simulink model "tempE"  (Simulink 6.1)
settings: Solver=ode3  StartTime=0.0  StopTime=5  FixedStep=0.1  RelTol=1e-3
libraries: simulink x5
settings Model: LastModifiedBy=okawa
settings DebuggingCC: SolverPrmCheckMsg=warning

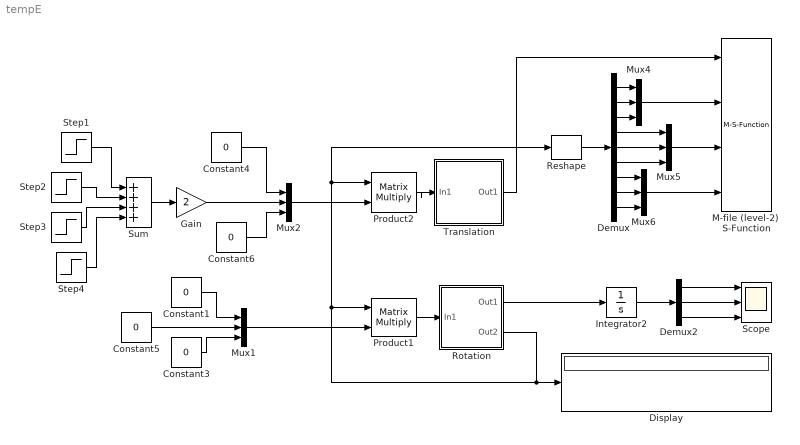
== system tempE ==
  Constant{1,3..6} (5 alike) : Constant  Value=0
  Demux : Demux  Outputs=9
  Demux2 : Demux  Outputs=3
  Display : Display
  Gain : Gain  Gain=2
  Integrator2 : Integrator
  M-file (level-2)  S-Function : M-S-Function  MFile=graphShip
  Mux{1..2,4..6} (5 alike) : Mux  Inputs=3
  Product1 : Product  Multiplication=Matrix(*)  RndMeth=Zero
  Product2 : Product  Multiplication=Matrix(*)  RndMeth=Zero
  Reshape : simulink/Math Operations/Reshape  OutputDimensionality=1-D array  OutputDimensions=[1,1]
  Rotation : Subsystem
  Scope : Scope  NumInputPorts=3
      settings: YMin=-5~-5~-5  YMax=5~5~5
  Step1 : Step  SampleTime=0
  Step2 : Step  Time=2  After=-2  SampleTime=0
  Step3 : Step  Time=4  After=2  SampleTime=0
  Step4 : Step  Time=5  After=-1  SampleTime=0
  Sum : Sum  Inputs=++++
  Translation : Subsystem
  wires:
  Demux/1 -> Mux4/1
  Demux/2 -> Mux4/2
  Demux/3 -> Mux4/3
  Demux/4 -> Mux5/1
  Demux/5 -> Mux5/2
  Demux/6 -> Mux5/3
  Demux/7 -> Mux6/1
  Demux/8 -> Mux6/2
  Demux/9 -> Mux6/3
  Rotation/1(Out1) -> Integrator2/1
  Rotation/2(Out2) -> Display/1, Product1/1, Reshape/1, Product2/1
  Product2/1 -> Translation/1(In1)
  Integrator2/1 -> Demux2/1
  Demux2/1 -> Scope/1
  Demux2/2 -> Scope/2
  Demux2/3 -> Scope/3
  Product1/1 -> Rotation/1(In1)
  Translation/1(Out1) -> M-file (level-2)  S-Function/1
  Reshape/1 -> Demux/1
  Mux2/1 -> Product2/2
  Step1/1 -> Sum/1
  Step2/1 -> Sum/2
  Step4/1 -> Sum/4
  Constant6/1 -> Mux2/3
  Step3/1 -> Sum/3
  Constant4/1 -> Mux2/1
  Sum/1 -> Gain/1
  Gain/1 -> Mux2/2
  Constant3/1 -> Mux1/3
  Constant5/1 -> Mux1/2
  Mux1/1 -> Product1/2
  Mux4/1 -> M-file (level-2)  S-Function/2
  Mux5/1 -> M-file (level-2)  S-Function/3
  Mux6/1 -> M-file (level-2)  S-Function/4
  Constant1/1 -> Mux1/1

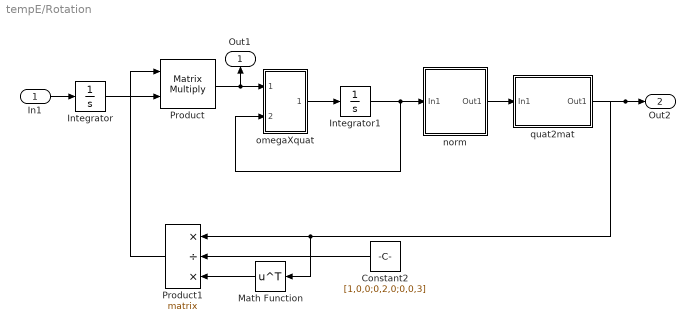
== system tempE/Rotation ==
  In1 : Inport  Port=1  LatchInput=off
  Constant2 : Constant  Orientation=left  Value=[1,0,0;0,2,0;0,0,3]  VectorParams1D=off
  Integrator : Integrator
  Integrator1 : Integrator  InitialCondition=[1;0;0;0]
  Math Function : Math  Orientation=left  Operator=transpose  SaturateOnIntegerOverflow=on
  Product : Product  Multiplication=Matrix(*)  RndMeth=Zero
  Product1 : Product  Orientation=left  Inputs=*/*  Multiplication=Matrix(*)  RndMeth=Zero
  norm : Subsystem
  "omegaXquat " : Subsystem
  quat2mat : Subsystem
  Out1 : Outport  Orientation=up
  Out2 : Outport  Port=2
  wires:
  Integrator/1 -> Product/2
  Product1/1 -> Product/1
  Product/1 -> "omegaXquat "/1(In1), Out1/1
  "omegaXquat "/1(Out1) -> Integrator1/1
  Integrator1/1 -> "omegaXquat "/2(In2), norm/1(In1)
  quat2mat/1(Out1) -> Product1/1, Math Function/1, Out2/1
  Constant2/1 -> Product1/2
  Math Function/1 -> Product1/3
  norm/1(Out1) -> quat2mat/1(In1)
  In1/1 -> Integrator/1

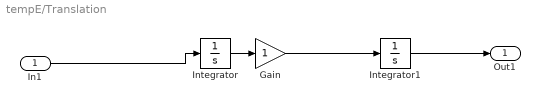
== system tempE/Translation ==
  In1 : Inport  Port=1  LatchInput=off
  Gain : Gain
  Integrator : Integrator
  Integrator1 : Integrator
  Out1 : Outport
  wires:
  Integrator/1 -> Gain/1
  Gain/1 -> Integrator1/1
  In1/1 -> Integrator/1
  Integrator1/1 -> Out1/1

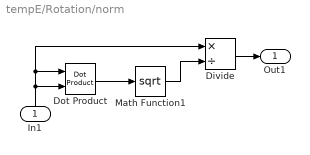
== system tempE/Rotation/norm ==
  In1 : Inport  Orientation=up  Port=1  LatchInput=off
  Divide : Product  Inputs=*/  OutScaling=2^-10
  Dot Product : simulink/Math Operations/Dot Product  InputSameDT=on  OutDataType=sfix(16)  OutScaling=2^-10  DoSatur=off
  Math Function1 : Math  Operator=sqrt  SaturateOnIntegerOverflow=on
  Out1 : Outport
  wires:
  Dot Product/1 -> Math Function1/1
  Math Function1/1 -> Divide/2
  In1/1 -> Dot Product/2, Dot Product/1, Divide/1
  Divide/1 -> Out1/1

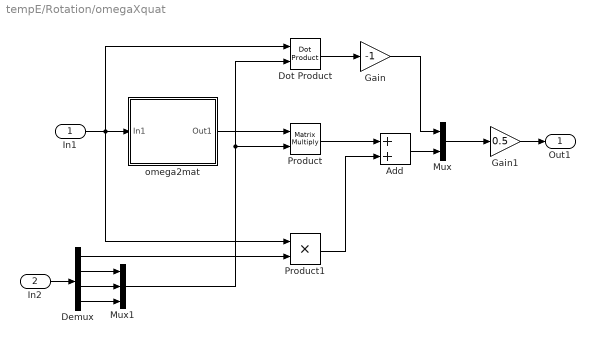
== system tempE/Rotation/omegaXquat  ==
  In1 : Inport  Port=1  LatchInput=off
  In2 : Inport  Port=2  LatchInput=off
  Add : Sum  OutScaling=2^-10
  Demux : Demux
  Dot Product : simulink/Math Operations/Dot Product  InputSameDT=on  OutDataType=sfix(16)  OutScaling=2^-10  DoSatur=off
  Gain : Gain  Gain=-1
  Gain1 : Gain  Gain=0.5
  Mux : Mux  Inputs=2
  Mux1 : Mux  Inputs=3
  Product : Product  Multiplication=Matrix(*)  RndMeth=Zero
  Product1 : Product  RndMeth=Zero
  omega2mat : Subsystem
  Out1 : Outport
  wires:
  In1/1 -> Product1/1, Dot Product/1, omega2mat/1(In1)
  Dot Product/1 -> Gain/1
  omega2mat/1(Out1) -> Product/1
  Product/1 -> Add/1
  Product1/1 -> Add/2
  Gain/1 -> Mux/1
  Add/1 -> Mux/2
  Mux/1 -> Gain1/1
  Demux/2 -> Mux1/1
  Demux/3 -> Mux1/2
  Demux/4 -> Mux1/3
  Mux1/1 -> Dot Product/2, Product/2
  Demux/1 -> Product1/2
  Gain1/1 -> Out1/1
  In2/1 -> Demux/1

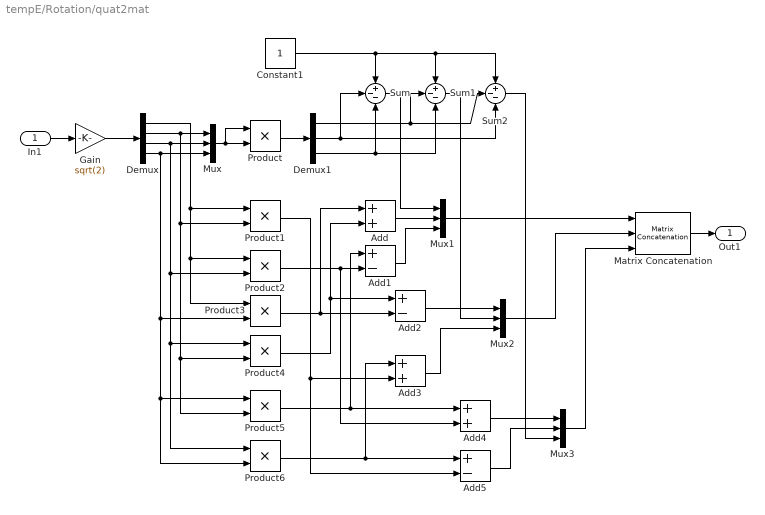
== system tempE/Rotation/quat2mat ==
  In1 : Inport  Port=1  LatchInput=off
  Add : Sum  OutScaling=2^-10
  Add1 : Sum  Inputs=+-  OutScaling=2^-10
  Add2 : Sum  Inputs=+-  OutScaling=2^-10
  Add3 : Sum  OutScaling=2^-10
  Add4 : Sum  OutScaling=2^-10
  Add5 : Sum  Inputs=+-  OutScaling=2^-10
  Constant1 : Constant
  Demux : Demux
  Demux1 : Demux  Outputs=3
  Gain : Gain  Gain=sqrt(2)
  Matrix Concatenation : simulink/Math Operations/Matrix Concatenation  numInports=3  catMethod=Horizontal
  Mux{,1..3} (4 alike) : Mux  Inputs=3
  Product{,1..6} (7 alike) : Product  RndMeth=Zero
  Sum : Sum  Inputs=+--
  Sum1 : Sum  Inputs=+--
  Sum2 : Sum  Inputs=+--
  Out1 : Outport
  wires:
  Gain/1 -> Demux/1
  Demux/2 -> Mux/1, Product1/2, Product5/2, Product4/2
  Demux/3 -> Mux/2, Product6/1, Product4/1, Product2/2
  Demux/4 -> Mux/3, Product6/2, Product5/1, Product3/2
  Mux/1 -> Product/2, Product/1
  Product/1 -> Demux1/1
  Constant1/1 -> Sum/1, Sum2/1, Sum1/1
  Demux1/1 -> Sum2/2, Sum1/2
  Demux1/2 -> Sum2/3, Sum/2
  Demux1/3 -> Sum1/3, Sum/3
  Demux/1 -> Product1/1, Product3/1, Product2/1
  Mux1/1 -> Matrix Concatenation/1
  Mux3/1 -> Matrix Concatenation/3
  Mux2/1 -> Matrix Concatenation/2
  Add4/1 -> Mux3/1
  Add5/1 -> Mux3/2
  Sum2/1 -> Mux3/3
  Product6/1 -> Add5/1, Add3/1
  Product1/1 -> Add5/2, Add3/2
  Product5/1 -> Add4/1, Add1/1
  Add2/1 -> Mux2/1
  Sum1/1 -> Mux2/2
  Add3/1 -> Mux2/3
  Sum/1 -> Mux1/1
  Add/1 -> Mux1/2
  Add1/1 -> Mux1/3
  Product3/1 -> Add2/2, Add/1
  Product4/1 -> Add/2, Add2/1
  Product2/1 -> Add1/2, Add4/2
  In1/1 -> Gain/1
  Matrix Concatenation/1 -> Out1/1

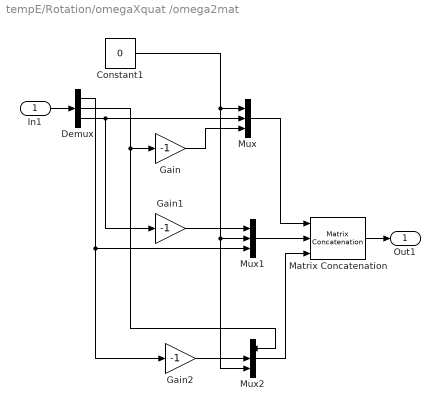
== system tempE/Rotation/omegaXquat /omega2mat ==
  In1 : Inport  Port=1  LatchInput=off
  Constant1 : Constant  Value=0
  Demux : Demux  Outputs=3
  Gain : Gain  Gain=-1
  Gain1 : Gain  Gain=-1
  Gain2 : Gain  Gain=-1
  Matrix Concatenation : simulink/Math Operations/Matrix Concatenation  numInports=3  catMethod=Horizontal
  Mux : Mux  Inputs=3
  Mux1 : Mux  Inputs=3
  Mux2 : Mux  Inputs=3
  Out1 : Outport
  wires:
  Constant1/1 -> Mux/1, Mux1/2, Mux2/3
  Demux/2 -> Gain/1, Mux2/1
  Gain/1 -> Mux/3
  Demux/3 -> Mux/2, Gain1/1
  Gain1/1 -> Mux1/1
  Demux/1 -> Mux1/3, Gain2/1
  Gain2/1 -> Mux2/2
  Mux/1 -> Matrix Concatenation/1
  Mux1/1 -> Matrix Concatenation/2
  Mux2/1 -> Matrix Concatenation/3
  In1/1 -> Demux/1
  Matrix Concatenation/1 -> Out1/1
